simulink model "end2end_control_view"  (R2014a)
settings: Solver=ode45  StartTime=0.0  StopTime=10.0  RelTol=1e-3
libraries: visionsinks x1, visiontextngfix x1
settings Model: Creator=Edward  LastModifiedBy=Administrator
settings DebuggingCC: MergeDetectMultiDrivingBlocksExec=error

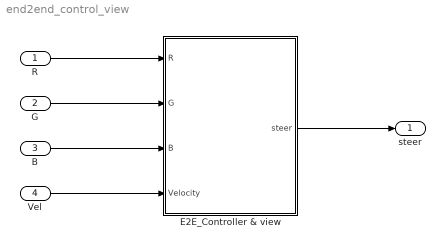
== system end2end_control_view ==
  R : Inport
  G : Inport  Port=2
  B : Inport  Port=3
  Vel : Inport  Port=4
  E2E_Controller & view : Subsystem
  steer : Outport
  wires:
  R/1 -> E2E_Controller & view/1(R)
  G/1 -> E2E_Controller & view/2(G)
  B/1 -> E2E_Controller & view/3(B)
  E2E_Controller & view/1(steer) -> steer/1
  Vel/1 -> E2E_Controller & view/4(Velocity)

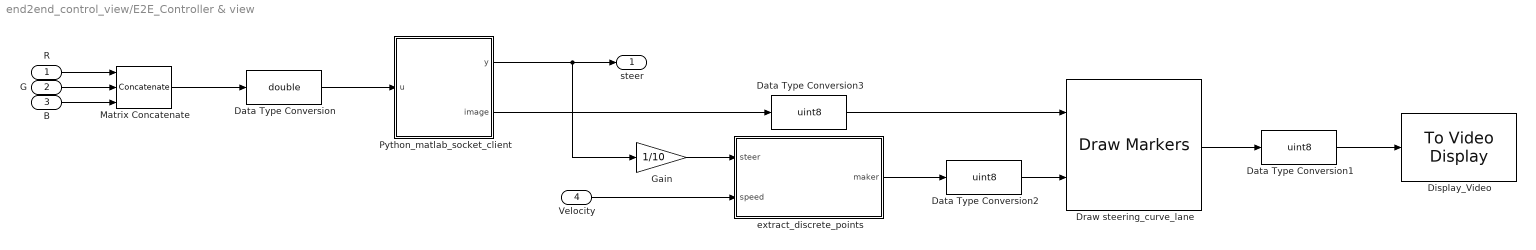
== system end2end_control_view/E2E_Controller & view ==
  R : Inport
  G : Inport  Port=2
  B : Inport  Port=3
  Velocity : Inport  Port=4
  Data Type Conversion : DataTypeConversion  OutDataTypeStr=double
  Data Type Conversion1 : DataTypeConversion  OutDataTypeStr=uint8
  Data Type Conversion2 : DataTypeConversion  OutDataTypeStr=uint8
  Data Type Conversion3 : DataTypeConversion  OutDataTypeStr=uint8
  Display_Video : visionsinks/To Video Display  inputType=Obsolete  imagePorts=One multidimensional signal  OutputDevice=On-screen video monitor  fullScreen=off  videoWindowX=258  videoWindowY=137  saveWindowSize=off  videoWindowWidth=360  videoWindowHeight=120  dataOrg=Column-major  openAtMdlStart=on  isWindowOpen=off  inputColorFormat=RGB
  Draw steering_curve_lane : visiontextngfix/Draw Markers  shape=Circle  size=1  fill=on  fillClrSource=Specify via dialog  display=User-specified value  intensity=200  color=[0 0 255]  opacity=0.6  viewport=Entire image  antialiasing=off  inType=Obsolete  imagePorts=One multidimensional signal  prodOutputMode=Binary point scaling  prodOutputWordLength=32  prodOutputFracLength=14  memoryMode=Specify word length  memoryWordLength=16  memoryFracLength=14  roundingMode=Floor  overflowMode=off
  Gain : Gain  Gain=1/10
  Matrix Concatenate : Concatenate  NumInputs=3  Mode=Multidimensional array  ConcatenateDimension=3
  Python_matlab_socket_client : MATLAB Function  TreatAsAtomicUnit=on
  extract_discrete_points : MATLAB Function  TreatAsAtomicUnit=on
  steer : Outport
  wires:
  B/1 -> Matrix Concatenate/3
  Data Type Conversion2/1 -> Draw steering_curve_lane/2
  Python_matlab_socket_client/2(image) -> Data Type Conversion3/1
  Data Type Conversion1/1 -> Display_Video/1
  Data Type Conversion/1 -> Python_matlab_socket_client/1(u)
  Gain/1 -> extract_discrete_points/1(steer)
  Velocity/1 -> extract_discrete_points/2(speed)
  extract_discrete_points/1(maker) -> Data Type Conversion2/1
  Python_matlab_socket_client/1(y) -> steer/1, Gain/1
  G/1 -> Matrix Concatenate/2
  Data Type Conversion3/1 -> Draw steering_curve_lane/1
  R/1 -> Matrix Concatenate/1
  Draw steering_curve_lane/1 -> Data Type Conversion1/1
  Matrix Concatenate/1 -> Data Type Conversion/1

== matlab function end2end_control_view/E2E_Controller & view/Python_matlab_socket_client ==
  data: u input; y output; image output
function [y,image]= fcn(u)
coder.extrinsic('tcpip')
coder.extrinsic('str2num')
coder.extrinsic('char')
coder.extrinsic('fwrite')
coder.extrinsic('imcrop')
t = tcpip('localhost',54322, 'Timeout', 1000, 'OutputBufferSize',1024);
fopen(t);
image = zeros(120,360,3);
image = imcrop(u,[150, 220, 359, 119]);
im = reshape(image, 129600,1);
buffer = uint8(im);
filesize = 129600;
nBytes = 0;
%header = 'start';
%fwrite(t,header); % 发送一段数据给tcp服务器，服务器知道matlab的ip和端口
send_size = 0;
while(1)
    if filesize-send_size >= 1024
        data = buffer(send_size+1:send_size + 1024) ;
        fwrite(t,data,'uint8'); % 发送一段数据给tcp服务器，服务器知道matlab的ip和端口
        send_size = send_size + 1024;
	elseif filesize-send_size>0 && filesize-send_size <1024
        data = buffer(send_size+1:filesize);
        fwrite(t,data,'uint8'); % 发送一段数据给tcp服务器，服务器知道matlab的ip和端口
        break;
    end
end
    %fprintf('%d\n', send_size);
%time1 = cputime;
while(1)
   % time2 = cputime;
	nBytes = get(t,'BytesAvailable');
    if nBytes > 0
        break;
    end
end
receive = fread(t,nBytes); %读取tcp服务器传来的数据
%fread(t);
fclose(t);
receive = char(receive');
steer = str2num(receive);%Ascaii码转换为str，再将str转换为数组
%fprintf('%f\n', steer);
y = 0;
y = steer;
end

== matlab function end2end_control_view/E2E_Controller & view/extract_discrete_points ==
  data: steer input; maker output; speed input
function maker = draw_path_on(steer,speed)
coder.extrinsic('cp2tform')
coder.extrinsic('Stuct')
coder.extrinsic('tformfwd')
path_x = 0: 0.5: 50;
angle_steers = steer;
v_ego = speed;
rsrc = [43.45456230828867, 118.00743250075844;
  104.5055617352614, 69.46865203761757;
  114.86050156739812, 60.83953551083698;
  129.74572757609468, 50.48459567870026;
  132.98164627363735, 46.38576532847949;
  301.0336906326895, 98.16046448916306;
  238.25686790036065, 62.56535881619311;
  227.2547443287154, 56.30924933427718;
  209.13359962247614, 46.817221154818526;
  203.9561297064078, 43.5813024572758];
rdst = [10.822125594094452, 1.42189132706374;
  21.177065426231174, 1.5297552836484982 ;
  25.275895776451954, 1.42189132706374;
  36.062291434927694, 1.6376192402332563;
  40.376849698318004, 1.42189132706374 ;
  11.900765159942026, -2.1376192402332563;
  22.25570499207874, -2.1376192402332563;
  26.785991168638553, -2.029755283648498;
 37.033067044190524, -2.029755283648498;
  41.67121717733509, -2.029755283648498];

%parameters
  H = [-0.0107277373418100,-36.7583251307781,160.036017000316;
      -1.98400305257070,1.43905526933179,119.918711008439;
      1.05534163114818e-17,-3.60414129149914e-18,1.00000000000000];
  deg_to_rad = pi/180.;
  slip_fator = 0.0014 ;
  steer_ratio = 10 ;
  wheel_base = 2.67 ;
  angle_offset = 0;
  angle_steers_rad = (angle_steers - angle_offset) * deg_to_rad;
  curvature = angle_steers_rad/(steer_ratio * wheel_base * (1. + slip_fator * v_ego^2));
  temp = zeros(1,101);
  temp = path_x .* curvature;
  for i = 1:1:101
      if temp(i)> 0.999
          temp(i) = 0.999;
      end
      if temp(i) <-0.999
          temp(i) = -0.999;
      end
  end
  y_actual = path_x .* tan(asin(temp)/2.)
  dst= zeros(101,2);
  maker = zeros(101,2);
  dst(:,1) = path_x;
  dst(:,2) = y_actual;
  TForm = cp2tform(rdst,rsrc,'projective');
  maker = round(tformfwd(TForm,dst));
  maker(:,1) = maker(:,1) + 20
end
